simulink model "ES200A_CurrMeas"  (R2013b)
settings: Solver=FixedStepDiscrete  SolverMode=SingleTasking  StartTime=0.0  StopTime=1  FixedStep=0.000125  RelTol=1e-3
values from neighbouring files (symbols this model uses):
  ARCHGLBPRM_2PI_ULS_F32 = DataDict.Constant    [ES200A_CurrMeas_DataDict.m]
  CurrMeasEolGainMax = DataDict.Calibration    [ES200A_CurrMeas_DataDict.m]
  CurrMeasEolGainMin = DataDict.Calibration    [ES200A_CurrMeas_DataDict.m]
  CurrMeasEolGainNrOfSample = DataDict.Calibration    [ES200A_CurrMeas_DataDict.m]
  CurrMeasEolGainNumer = DataDict.Calibration    [ES200A_CurrMeas_DataDict.m]
  CurrMeasEolMaxMotVel = DataDict.Calibration    [ES200A_CurrMeas_DataDict.m]
  CurrMeasEolOffsHiBrdgVltgMin = DataDict.Calibration    [ES200A_CurrMeas_DataDict.m]
  CurrMeasEolOffsHiCmuOffs = DataDict.Calibration    [ES200A_CurrMeas_DataDict.m]
  CurrMeasEolOffsLoCmuOffs = DataDict.Calibration    [ES200A_CurrMeas_DataDict.m]
  CurrMeasEolOffsMax = DataDict.Calibration    [ES200A_CurrMeas_DataDict.m]
  CurrMeasEolOffsMin = DataDict.Calibration    [ES200A_CurrMeas_DataDict.m]
  CurrMeasEolOffsNrOfSample = DataDict.Calibration    [ES200A_CurrMeas_DataDict.m]
  CurrMeasEolTranCntrThd = DataDict.Calibration    [ES200A_CurrMeas_DataDict.m]
  CurrMeasMinRqrdPhaOnTi = DataDict.Calibration    [ES200A_CurrMeas_DataDict.m]
  CurrMeasMotAgCompuDly = DataDict.Calibration    [ES200A_CurrMeas_DataDict.m]
  CurrMeasMotCurrAdcVlyWrmIninMax = DataDict.Calibration    [ES200A_CurrMeas_DataDict.m]
  CurrMeasMotCurrAdcVlyWrmIninMin = DataDict.Calibration    [ES200A_CurrMeas_DataDict.m]
  CurrMeasNtc0x05DFailStep = DataDict.Calibration    [ES200A_CurrMeas_DataDict.m]
  CurrMeasNtc0x05DPassStep = DataDict.Calibration    [ES200A_CurrMeas_DataDict.m]
  CurrMeasNtc0x06DFailStep = DataDict.Calibration    [ES200A_CurrMeas_DataDict.m]
  CurrMeasNtc0x06DPassStep = DataDict.Calibration    [ES200A_CurrMeas_DataDict.m]
  DEGREES30_MOTRAD_F32 = DataDict.Constant    [ES200A_CurrMeas_DataDict.m]
  DIFOFFSRNGCHKMAX_VOLT_F32 = DataDict.Constant    [ES200A_CurrMeas_DataDict.m]
  ELECGLBPRM_IVTRCNT_CNT_U08 = DataDict.ConfigParam    [ES200A_CurrMeas_DataDict.m]
  ELECGLBPRM_STRTUPSTCURRMEASWRMININTESTSTRT_CNT_U08 = DataDict.Constant    [ES200A_CurrMeas_DataDict.m]
  FLTINJ_CURRMEAS_MOTCURRCORRDA = DataDict.Constant    [ES200A_CurrMeas_DataDict.m]
  FLTINJ_CURRMEAS_MOTCURRCORRDD = DataDict.Constant    [ES200A_CurrMeas_DataDict.m]
  FLTINJ_CURRMEAS_TESTOK = DataDict.Constant    [ES200A_CurrMeas_DataDict.m]
  MAXCURRCORRD_AMPR_F32 = DataDict.Constant    [ES200A_CurrMeas_DataDict.m]
  PhaABCMeasdOutOfRng = DataDict.NTC    [ES200A_CurrMeas_DataDict.m]
  PhaDEFMeasOutOfRng = DataDict.NTC    [ES200A_CurrMeas_DataDict.m]
  SysGlbPrmMotPoleCnt = DataDict.ImprtdCal    [ES200A_CurrMeas_DataDict.m]
libraries: simulink x10, FixdToFloat x1
(part 4 of 7)

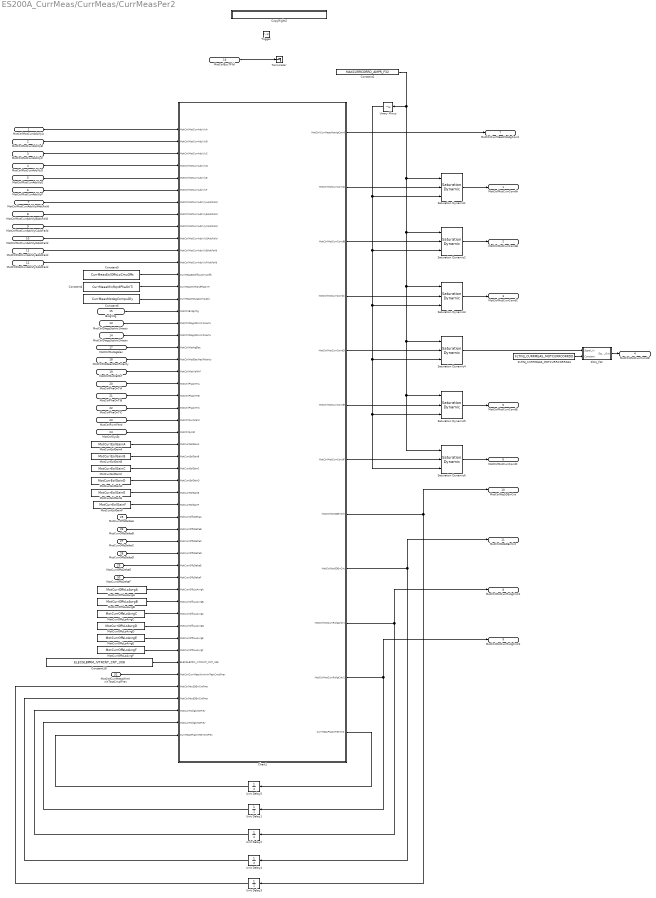
== system ES200A_CurrMeas/CurrMeas/CurrMeasPer2 ==
  MotCtrlMotCurrAdcVlyA : Inport  RequirementInfo={} %GIDa_51523d33_6191_4b88_8694_817dc9ded571
  MotCtrlMotCurrAdcVlyB : Inport  RequirementInfo={} %GIDa_1328ae42_ae96_4bf4_89b7_7635d71eb55f  Port=2
  MotCtrlMotCurrAdcVlyC : Inport  RequirementInfo={} %GIDa_141aa39a_2219_4c7a_8648_7879c9127c56  Port=3
  MotCtrlMotCurrAdcVlyD : Inport  RequirementInfo={} %GIDa_0bb8dbbc_c7c5_4117_b4a1_ced2a35897c9  Port=4
  MotCtrlMotCurrAdcVlyE : Inport  RequirementInfo={} %GIDa_e7be49ef_22f9_4690_b020_08185c31c438  Port=5
  MotCtrlMotCurrAdcVlyF : Inport  RequirementInfo={} %GIDa_885c6b45_efc1_4125_8826_e1fe2f9bfc98  Port=6
  MotCtrlMotCurrAdcVlyAAdcFaild : Inport  RequirementInfo={} %GIDa_d667bfad_9ccb_4ad0_ab64_59c5adeb3cfc  Port=7
  MotCtrlMotCurrAdcVlyBAdcFaild : Inport  RequirementInfo={} %GIDa_614f9520_457f_4a4d_a608_e6a9d7384c30  Port=8
  MotCtrlMotCurrAdcVlyCAdcFaild : Inport  RequirementInfo={} %GIDa_26dea516_d730_426b_b0f7_aef164a4b4a7  Port=9
  MotCtrlMotCurrAdcVlyDAdcFaild : Inport  RequirementInfo={} %GIDa_a9ef4412_4995_4ff8_a712_a0004978e7c0  Port=10
  MotCtrlMotCurrAdcVlyEAdcFaild : Inport  RequirementInfo={} %GIDa_8c5e2e43_d825_49af_8c14_bb63c0e12ba2  Port=11
  MotCtrlMotCurrAdcVlyFAdcFaild : Inport  RequirementInfo={} %GIDa_7ba5334c_0964_494c_9a84_9ee8fa4a837c  Port=12
  MotCtrlDiagcStsIvtr1Inactv : Inport  Port=13
  MotCtrlDiagcStsIvtr2Inactv : Inport  Port=14
  BrdgVltg : Inport  Port=15
  MotCtrlEcuTFild : Inport  RequirementInfo={} %GIDa_37deaa24_f58f_4dab_941a_680d37588f61  Port=16
  MotCtrlMotAgElec : Inport  Port=17
  MotCtrlMotElecMeclPolarity : Inport  Port=18
  MotCtrlMotVelMrf : Inport  Port=19
  MotCtrlPhaOnTiA : Inport  Port=20
  MotCtrlPhaOnTiB : Inport  Port=21
  MotCtrlPhaOnTiC : Inport  Port=22
  MotCtrlPwmPerd : Inport  Port=23
  MotCtrlSysSt : Inport  Port=24
  MotCurrOffsDeltaA : Inport  Port=25
  MotCurrOffsDeltaB : Inport  Port=26
  MotCurrOffsDeltaC : Inport  Port=27
  MotCurrOffsDeltaD : Inport  Port=28
  MotCurrOffsDeltaE : Inport  Port=29
  MotCurrOffsDeltaF : Inport  Port=30
  " MotCtrlCurrMeasWrmIninTestCmplPrev" : Inport  Port=31
  Trigger : TriggerPort  TriggerType=function-call  PortDimensions=1
  Chart1 : Stateflow chart  RequirementInfo={} %GIDa_9666b06e_9e22_4012_a59d_551b4af1f380  TreatAsAtomicUnit=on
  Constant18 : Constant  Value=ELECGLBPRM_IVTRCNT_CNT_U08
  Constant2 : Constant  Value=MAXCURRCORRD_AMPR_F32
  Constant4 : Constant  Value=CurrMeasMinRqrdPhaOnTi
  Constant5 : Constant  Value=CurrMeasEolOffsLoCmuOffs
  Constant6 : Constant  Value=CurrMeasMotAgCompuDly
  CopyRight2 : Subsystem  Description=|  mask(Copyright Information){none=on}
      | Copyright info block.                                               
      |                                                                     
      | Place copyright information at the top of every subsystem in design.
      mask prompts: none "No parameters"
      mask help: Place copyright information at the top of every subsystem in design.
      mask Display:
      | NxtrConf = 'Nexteer Confidential';
      | 
      | sys = bdroot; %handle for the current model ("system")
      | first = get_param(sys,'Created');
      | first = first(end-3:end);  %year is last four digits
      | 
      | last = get_param(sys,'LastModifiedDate');
      | if isempty(last)
      |     last = datestr(now,'yyyy');
      | else
      |     last = last(end-3:end);
      | end
      | 
      | if strcmp(first,last)
      |     fprintf('%s -- Copyright %s Nexteer',NxtrConf,first)
      | else
      |     fprintf('%s -- %s%s- %s Nexteer',NxtrConf,char(169),first,last)
      | end
  FLTINJ_CURRMEAS_MOTCURRCORRDA1 : Constant  Value=FLTINJ_CURRMEAS_MOTCURRCORRDD
  FltInj_f32 : Subsystem  RequirementInfo={'linktype_rmi_doors' '000089bc (/ESG Group/FDD Module Requirements/EA4 Specific/ES200A_CurrMeas)' '#ES200A_267' 'true' 'REQ: ES200A_267' '' } %GIDa_347b8ae7_8767_40c8_a00c_71aafa320d2d  TreatAsAtomicUnit=on  VariantControl=FltInj_sim  mask(Fault_Injection){}
      mask help: Fault Injection is a simulation only block for EA3 programs.
  MotCurrEolGainA : DataStoreRead  DataStoreName=MotCurrEolGainA
  MotCurrEolGainB : DataStoreRead  DataStoreName=MotCurrEolGainB
  MotCurrEolGainC : DataStoreRead  DataStoreName=MotCurrEolGainC
  MotCurrEolGainD : DataStoreRead  DataStoreName=MotCurrEolGainD
  MotCurrEolGainE : DataStoreRead  DataStoreName=MotCurrEolGainE
  MotCurrEolGainF : DataStoreRead  DataStoreName=MotCurrEolGainF
  MotCurrOffsLoAvrgA : DataStoreRead  DataStoreName=MotCurrOffsLoAvrgA
  MotCurrOffsLoAvrgB : DataStoreRead  DataStoreName=MotCurrOffsLoAvrgB
  MotCurrOffsLoAvrgC : DataStoreRead  DataStoreName=MotCurrOffsLoAvrgC
  MotCurrOffsLoAvrgD : DataStoreRead  DataStoreName=MotCurrOffsLoAvrgD
  MotCurrOffsLoAvrgE : DataStoreRead  DataStoreName=MotCurrOffsLoAvrgE
  MotCurrOffsLoAvrgF : DataStoreRead  DataStoreName=MotCurrOffsLoAvrgF
  Saturation Dynamic1 : simulink/Discontinuities/Saturation Dynamic  RequirementInfo={} %GIDa_a678ac9c_94e0_45a6_bd24_feb3ddad182c  OutMin=[]  OutMax=[]  OutDataTypeStr=Inherit: Same as second input  OutDataType=fixdt(1, 16)  OutScaling=2^-10  DoSatur=off
  Saturation Dynamic2 : simulink/Discontinuities/Saturation Dynamic  RequirementInfo={} %GIDa_ad27d5c1_4180_4794_bb6c_e90600e03b36  OutMin=[]  OutMax=[]  OutDataTypeStr=Inherit: Same as second input  OutDataType=fixdt(1, 16)  OutScaling=2^-10  DoSatur=off
  Saturation Dynamic3 : simulink/Discontinuities/Saturation Dynamic  RequirementInfo={} %GIDa_b6946fe3_e777_41d1_91e9_ba0e49afc616  OutMin=[]  OutMax=[]  OutDataTypeStr=Inherit: Same as second input  OutDataType=fixdt(1, 16)  OutScaling=2^-10  DoSatur=off
  Saturation Dynamic4 : simulink/Discontinuities/Saturation Dynamic  RequirementInfo={} %GIDa_eac887ff_7631_462d_b878_5019172b3d55  OutMin=[]  OutMax=[]  OutDataTypeStr=Inherit: Same as second input  OutDataType=fixdt(1, 16)  OutScaling=2^-10  DoSatur=off
  Saturation Dynamic5 : simulink/Discontinuities/Saturation Dynamic  RequirementInfo={} %GIDa_d9181953_bf05_4f89_9278_4fcbc01ab15c  OutMin=[]  OutMax=[]  OutDataTypeStr=Inherit: Same as second input  OutDataType=fixdt(1, 16)  OutScaling=2^-10  DoSatur=off
  Saturation Dynamic6 : simulink/Discontinuities/Saturation Dynamic  RequirementInfo={} %GIDa_4da0401d_6120_4b21_aef3_0a502043331b  OutMin=[]  OutMax=[]  OutDataTypeStr=Inherit: Same as second input  OutDataType=fixdt(1, 16)  OutScaling=2^-10  DoSatur=off
  Terminator : Terminator
  Unary Minus : UnaryMinus
  Unit Delay1 : UnitDelay  SampleTime=-1  StateName=MotCurrRollgCnt2Prev  StateMustResolveToSignalObject=on
      settings: AttributesFormatString=|
      | State Variable:
      | %<StateName>
  Unit Delay2 : UnitDelay  SampleTime=-1  StateName=MotCurrRollgCnt1Prev  StateMustResolveToSignalObject=on
      settings: AttributesFormatString=|
      | State Variable:
      | %<StateName>
  Unit Delay3 : UnitDelay  SampleTime=-1  StateName=MotCtrlNtc5DErrCntPrev  StateMustResolveToSignalObject=on
      settings: AttributesFormatString=|
      | State Variable:
      | %<StateName>
  Unit Delay4 : UnitDelay  SampleTime=-1  StateName=MotCtrlNtc6DErrCntPrev  StateMustResolveToSignalObject=on
      settings: AttributesFormatString=|
      | State Variable:
      | %<StateName>
  Unit Delay5 : UnitDelay  SampleTime=-1  StateName=PhaOnTiErrCntPrev  StateMustResolveToSignalObject=on
      settings: AttributesFormatString=|
      | State Variable:
      | %<StateName>
  MotCtrlMotCurrCorrdA : Outport  RequirementInfo={} %GIDa_be45cc68_c253_4805_9e57_9f0cd86a4b75
  MotCtrlMotCurrCorrdB : Outport  RequirementInfo={} %GIDa_38a03b4c_0b98_4645_8602_2d424e547661  Port=2
  MotCtrlMotCurrCorrdC : Outport  RequirementInfo={} %GIDa_14a10ace_ee81_4ce4_9336_8f01f385929c  Port=3
  MotCtrlMotCurrCorrdD : Outport  RequirementInfo={} %GIDa_2faaf7ab_4344_43ac_a199_98727489f260  Port=4
  MotCtrlMotCurrCorrdE : Outport  RequirementInfo={} %GIDa_8650b4b3_021a_4514_9f56_5151faf8a566  Port=5
  MotCtrlMotCurrCorrdF : Outport  RequirementInfo={} %GIDa_2593a86b_f65b_45be_b765_d74bea967e23  Port=6
  MotCtrlCurrMeasMotAgCorrd : Outport  RequirementInfo={} %GIDa_90a95302_1bff_47e7_a89a_896fae3a575d  Port=7
  MotCtrlMotCurrRollgCntr1 : Outport  RequirementInfo={} %GIDa_aefa170b_455b_48cb_95aa_73c7254f08bd  Port=8
  MotCtrlMotCurrRollgCntr2 : Outport  RequirementInfo={} %GIDa_b45ba8e0_1343_4e05_96b1_238e41ca7131  Port=9
  MotCtrlNtc5DErrCnt : Outport  RequirementInfo={} %GIDa_6d95d8c9_c06f_4998_9e76_5195a73bd44f  Port=10
  MotCtrlNtc6DErrCnt : Outport  RequirementInfo={} %GIDa_f3d2e981_43dc_4e53_81d4_c9088f8342fd  Port=11
  wires:
  MotCtrlEcuTFild/1 -> Terminator/1
  MotCtrlMotCurrAdcVlyAAdcFaild/1 -> Chart1/7(MotCtrlMotCurrAdcVlyAAdcFaild)
  MotCtrlMotCurrAdcVlyBAdcFaild/1 -> Chart1/8(MotCtrlMotCurrAdcVlyBAdcFaild)
  MotCtrlMotCurrAdcVlyDAdcFaild/1 -> Chart1/10(MotCtrlMotCurrAdcVlyDAdcFaild)
  MotCtrlMotCurrAdcVlyFAdcFaild/1 -> Chart1/12(MotCtrlMotCurrAdcVlyFAdcFaild)
  MotCtrlMotCurrAdcVlyEAdcFaild/1 -> Chart1/11(MotCtrlMotCurrAdcVlyEAdcFaild)
  MotCtrlMotCurrAdcVlyCAdcFaild/1 -> Chart1/9(MotCtrlMotCurrAdcVlyCAdcFaild)
  Saturation Dynamic1/1 -> MotCtrlMotCurrCorrdA/1
  FltInj_f32/1(Signal_Out) -> MotCtrlMotCurrCorrdD/1
  FLTINJ_CURRMEAS_MOTCURRCORRDA1/1 -> FltInj_f32/2(Constant)
  Constant4/1 -> Chart1/14(CurrMeasMinRqrdPhaOnTi)
  Constant5/1 -> Chart1/13(CurrMeasEolOffsLoCmuOffs)
  Constant6/1 -> Chart1/15(CurrMeasMotAgCompuDly)
  MotCtrlMotVelMrf/1 -> Chart1/21(MotCtrlMotVelMrf)
  MotCtrlMotElecMeclPolarity/1 -> Chart1/20(MotCtrlMotElecMeclPolarity)
  BrdgVltg/1 -> Chart1/16(MotCtrlBrdgVltg)
  MotCtrlDiagcStsIvtr1Inactv/1 -> Chart1/17(MotCtrlDiagcStsIvtr1Inactv)
  MotCtrlDiagcStsIvtr2Inactv/1 -> Chart1/18(MotCtrlDiagcStsIvtr2Inactv)
  Constant18/1 -> Chart1/45(ELECGLBPRM_IVTRCNT_CNT_U08)
  Unit Delay1/1 -> Chart1/50(MotCurrRollgCnt2Prev)
  Unit Delay2/1 -> Chart1/49(MotCurrRollgCnt1Prev)
  Saturation Dynamic4/1 -> FltInj_f32/1(Signal_In)
  Saturation Dynamic2/1 -> MotCtrlMotCurrCorrdB/1
  Saturation Dynamic3/1 -> MotCtrlMotCurrCorrdC/1
  Saturation Dynamic5/1 -> MotCtrlMotCurrCorrdE/1
  Saturation Dynamic6/1 -> MotCtrlMotCurrCorrdF/1
  Chart1/10(MotCtrlMotCurrRollgCntr1) -> MotCtrlMotCurrRollgCntr1/1, Unit Delay2/1
  Chart1/11(MotCtrlMotCurrRollgCntr2) -> MotCtrlMotCurrRollgCntr2/1, Unit Delay1/1
  Chart1/1(MotCtrlCurrMeasMotAgCorrd) -> MotCtrlCurrMeasMotAgCorrd/1
  MotCurrOffsLoAvrgB/1 -> Chart1/40(MotCurrOffsLoAvrgB)
  MotCurrOffsLoAvrgA/1 -> Chart1/39(MotCurrOffsLoAvrgA)
  MotCurrOffsLoAvrgD/1 -> Chart1/42(MotCurrOffsLoAvrgD)
  MotCurrOffsLoAvrgC/1 -> Chart1/41(MotCurrOffsLoAvrgC)
  MotCurrOffsLoAvrgF/1 -> Chart1/44(MotCurrOffsLoAvrgF)
  MotCurrOffsLoAvrgE/1 -> Chart1/43(MotCurrOffsLoAvrgE)
  MotCurrEolGainF/1 -> Chart1/32(MotCurrEolGainF)
  MotCurrEolGainD/1 -> Chart1/30(MotCurrEolGainD)
  MotCurrEolGainE/1 -> Chart1/31(MotCurrEolGainE)
  MotCurrEolGainB/1 -> Chart1/28(MotCurrEolGainB)
  MotCurrEolGainC/1 -> Chart1/29(MotCurrEolGainC)
  MotCurrEolGainA/1 -> Chart1/27(MotCurrEolGainA)
  MotCurrOffsDeltaD/1 -> Chart1/36(MotCurrOffsDeltaD)
  MotCurrOffsDeltaC/1 -> Chart1/35(MotCurrOffsDeltaC)
  MotCtrlPhaOnTiC/1 -> Chart1/24(MotCtrlPhaOnTiC)
  MotCtrlSysSt/1 -> Chart1/26(MotCtrlSysSt)
  MotCtrlPwmPerd/1 -> Chart1/25(MotCtrlPwmPerd)
  MotCtrlPhaOnTiB/1 -> Chart1/23(MotCtrlPhaOnTiB)
  MotCurrOffsDeltaE/1 -> Chart1/37(MotCurrOffsDeltaE)
  MotCtrlPhaOnTiA/1 -> Chart1/22(MotCtrlPhaOnTiA)
  MotCurrOffsDeltaF/1 -> Chart1/38(MotCurrOffsDeltaF)
  MotCurrOffsDeltaA/1 -> Chart1/33(MotCurrOffsDeltaA)
  MotCurrOffsDeltaB/1 -> Chart1/34(MotCurrOffsDeltaB)
  Unit Delay4/1 -> Chart1/48(MotCtrlNtc6DErrCntPrev)
  Unit Delay3/1 -> Chart1/47(MotCtrlNtc5DErrCntPrev)
  Chart1/9(MotCtrlNtc6DErrCnt) -> MotCtrlNtc6DErrCnt/1, Unit Delay4/1
  Chart1/8(MotCtrlNtc5DErrCnt) -> MotCtrlNtc5DErrCnt/1, Unit Delay3/1
  " MotCtrlCurrMeasWrmIninTestCmplPrev"/1 -> Chart1/46(MotCtrlCurrMeasWrmIninTestCmplPrev)
  Unit Delay5/1 -> Chart1/51(CurrMeasPhaOnTiErrCntPrev)
  Chart1/12(CurrMeasPhaOnTiErrCnt) -> Unit Delay5/1
  Constant2/1 -> Saturation Dynamic3/1, Saturation Dynamic6/1, Saturation Dynamic5/1, Saturation Dynamic4/1, Saturation Dynamic2/1, Saturation Dynamic1/1, Unary Minus/1
  Unary Minus/1 -> Saturation Dynamic3/3, Saturation Dynamic6/3, Saturation Dynamic5/3, Saturation Dynamic4/3, Saturation Dynamic2/3, Saturation Dynamic1/3
  Chart1/2(MotCtrlMotCurrCorrdA) -> Saturation Dynamic1/2
  Chart1/3(MotCtrlMotCurrCorrdB) -> Saturation Dynamic2/2
  Chart1/4(MotCtrlMotCurrCorrdC) -> Saturation Dynamic3/2
  Chart1/5(MotCtrlMotCurrCorrdD) -> Saturation Dynamic4/2
  Chart1/6(MotCtrlMotCurrCorrdE) -> Saturation Dynamic5/2
  Chart1/7(MotCtrlMotCurrCorrdF) -> Saturation Dynamic6/2
  MotCtrlMotAgElec/1 -> Chart1/19(MotCtrlMotAgElec)
  MotCtrlMotCurrAdcVlyE/1 -> Chart1/5(MotCtrlMotCurrAdcVlyE)
  MotCtrlMotCurrAdcVlyD/1 -> Chart1/4(MotCtrlMotCurrAdcVlyD)
  MotCtrlMotCurrAdcVlyB/1 -> Chart1/2(MotCtrlMotCurrAdcVlyB)
  MotCtrlMotCurrAdcVlyC/1 -> Chart1/3(MotCtrlMotCurrAdcVlyC)
  MotCtrlMotCurrAdcVlyF/1 -> Chart1/6(MotCtrlMotCurrAdcVlyF)
  MotCtrlMotCurrAdcVlyA/1 -> Chart1/1(MotCtrlMotCurrAdcVlyA)

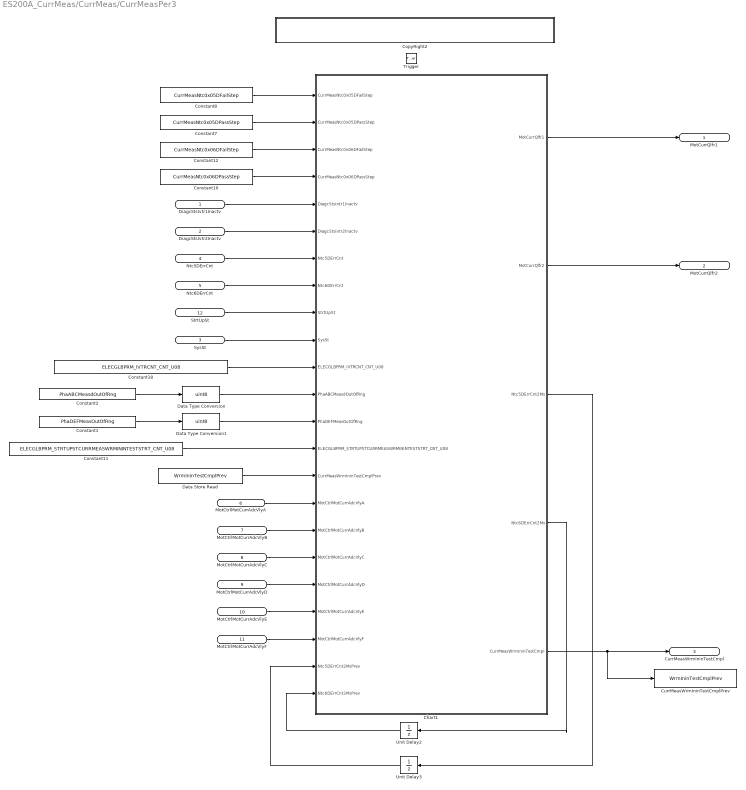
== system ES200A_CurrMeas/CurrMeas/CurrMeasPer3 ==
  DiagcStsIvtr1Inactv : Inport  RequirementInfo={} %GIDa_3f2b24ca_5e64_4642_910e_ca50d78da245
  DiagcStsIvtr2Inactv : Inport  RequirementInfo={} %GIDa_b1a5f59d_5a54_42de_8529_fc0d027b3ef3  Port=2
  SysSt : Inport  RequirementInfo={} %GIDa_ebc52ed6_1f51_43d3_a6da_39b6b9940c04  Port=3  OutDataTypeStr=single
  Ntc5DErrCnt : Inport  RequirementInfo={} %GIDa_ffc53944_d65d_4434_9c9b_5bfc70525927  Port=4  OutDataTypeStr=uint16
  Ntc6DErrCnt : Inport  RequirementInfo={} %GIDa_365cbd76_0dca_48e8_96f7_4dd33cc79fcb  Port=5  OutDataTypeStr=uint16
  MotCtrlMotCurrAdcVlyA : Inport  RequirementInfo={} %GIDa_7bf3cbd7_2538_4e8a_a22d_abe526b19335  Port=6
  MotCtrlMotCurrAdcVlyB : Inport  RequirementInfo={} %GIDa_7698553c_2590_423a_a37b_077079574e3f  Port=7
  MotCtrlMotCurrAdcVlyC : Inport  RequirementInfo={} %GIDa_493e93c2_e8a9_4c58_98a0_ce115796497b  Port=8
  MotCtrlMotCurrAdcVlyD : Inport  RequirementInfo={} %GIDa_dcf6e783_ea97_45aa_b2df_a8b40ffd71d9  Port=9
  MotCtrlMotCurrAdcVlyE : Inport  RequirementInfo={} %GIDa_a4c14b22_ad3d_4d49_8f67_e25589a32bce  Port=10
  MotCtrlMotCurrAdcVlyF : Inport  RequirementInfo={} %GIDa_1f7c68b9_6400_46f6_8cd6_6a391c1de49a  Port=11
  StrtUpSt : Inport  RequirementInfo={} %GIDa_1f30c06a_d58b_4090_b4a6_84109da18cdc  Port=12  OutDataTypeStr=single
  Trigger : TriggerPort  TriggerType=function-call  PortDimensions=1
  Chart1 : Stateflow chart  TreatAsAtomicUnit=on
  Constant1 : Constant  Value=PhaDEFMeasOutOfRng
  Constant10 : Constant  Value=CurrMeasNtc0x06DPassStep
  Constant11 : Constant  Value=ELECGLBPRM_STRTUPSTCURRMEASWRMININTESTSTRT_CNT_U08
  Constant12 : Constant  Value=CurrMeasNtc0x06DFailStep
  Constant18 : Constant  Value=ELECGLBPRM_IVTRCNT_CNT_U08
  Constant2 : Constant  Value=PhaABCMeasdOutOfRng
  Constant7 : Constant  Value=CurrMeasNtc0x05DPassStep
  Constant8 : Constant  Value=CurrMeasNtc0x05DFailStep
  CopyRight2 : Subsystem  Description=|  mask(Copyright Information){none=on}
      | Copyright info block.                                               
      |                                                                     
      | Place copyright information at the top of every subsystem in design.
      mask prompts: none "No parameters"
      mask help: Place copyright information at the top of every subsystem in design.
      mask Display:
      | NxtrConf = 'Nexteer Confidential';
      | 
      | sys = bdroot; %handle for the current model ("system")
      | first = get_param(sys,'Created');
      | first = first(end-3:end);  %year is last four digits
      | 
      | last = get_param(sys,'LastModifiedDate');
      | if isempty(last)
      |     last = datestr(now,'yyyy');
      | else
      |     last = last(end-3:end);
      | end
      | 
      | if strcmp(first,last)
      |     fprintf('%s -- Copyright %s Nexteer',NxtrConf,first)
      | else
      |     fprintf('%s -- %s%s- %s Nexteer',NxtrConf,char(169),first,last)
      | end
  CurrMeasWrmIninTestCmplPrev : DataStoreWrite  RequirementInfo={} %GIDa_56301e73_d1a5_44f0_9c00_c95c5be8192d  DataStoreName=WrmIninTestCmplPrev  DataStoreElements=WrmIninTestCmplPrev
  Data Store Read : DataStoreRead  DataStoreName=WrmIninTestCmplPrev  DataStoreElements=WrmIninTestCmplPrev
  Data Type Conversion : DataTypeConversion  OutDataTypeStr=uint8
  Data Type Conversion1 : DataTypeConversion  OutDataTypeStr=uint8
  Unit Delay2 : UnitDelay  SampleTime=-1  StateName=Ntc6DErrCnt2MilliSecPrev  StateMustResolveToSignalObject=on
      settings: AttributesFormatString=|
      | State Variable:
      | %<StateName>
  Unit Delay3 : UnitDelay  SampleTime=-1  StateName=Ntc5DErrCnt2MilliSecPrev  StateMustResolveToSignalObject=on
      settings: AttributesFormatString=|
      | State Variable:
      | %<StateName>
  MotCurrQlfr1 : Outport  RequirementInfo={} %GIDa_97d5bfb1_2351_42dd_b658_023a6d8f5aa1
  MotCurrQlfr2 : Outport  RequirementInfo={} %GIDa_e2da2e04_5849_4da3_a687_01333d2236a2  Port=2
  CurrMeasWrmIninTestCmpl : Outport  RequirementInfo={} %GIDa_b01ce9a2_2e51_43fa_ab76_6aeab0dbecf7  Port=3
  wires:
  Constant10/1 -> Chart1/4(CurrMeasNtc0x06DPassStep)
  Constant7/1 -> Chart1/2(CurrMeasNtc0x05DPassStep)
  Constant12/1 -> Chart1/3(CurrMeasNtc0x06DFailStep)
  Constant8/1 -> Chart1/1(CurrMeasNtc0x05DFailStep)
  DiagcStsIvtr1Inactv/1 -> Chart1/5(DiagcStsIvtr1Inactv)
  DiagcStsIvtr2Inactv/1 -> Chart1/6(DiagcStsIvtr2Inactv)
  Ntc5DErrCnt/1 -> Chart1/7(Ntc5DErrCnt)
  Ntc6DErrCnt/1 -> Chart1/8(Ntc6DErrCnt)
  Constant18/1 -> Chart1/11(ELECGLBPRM_IVTRCNT_CNT_U08)
  Constant11/1 -> Chart1/14(ELECGLBPRM_STRTUPSTCURRMEASWRMININTESTSTRT_CNT_U08)
  SysSt/1 -> Chart1/10(SysSt)
  Chart1/3(Ntc5DErrCnt2Ms) -> Unit Delay3/1
  Chart1/4(Ntc6DErrCnt2Ms) -> Unit Delay2/1
  Chart1/5(CurrMeasWrmIninTestCmpl) -> CurrMeasWrmIninTestCmpl/1, CurrMeasWrmIninTestCmplPrev/1
  Chart1/1(MotCurrQlfr1) -> MotCurrQlfr1/1
  Chart1/2(MotCurrQlfr2) -> MotCurrQlfr2/1
  Unit Delay2/1 -> Chart1/23(Ntc6DErrCnt2MsPrev)
  Unit Delay3/1 -> Chart1/22(Ntc5DErrCnt2MsPrev)
  Data Store Read/1 -> Chart1/15(CurrMeasWrmIninTestCmplPrev)
  Constant1/1 -> Data Type Conversion1/1
  Constant2/1 -> Data Type Conversion/1
  Data Type Conversion/1 -> Chart1/12(PhaABCMeasdOutOfRng)
  Data Type Conversion1/1 -> Chart1/13(PhaDEFMeasOutOfRng)
  MotCtrlMotCurrAdcVlyA/1 -> Chart1/16(MotCtrlMotCurrAdcVlyA)
  MotCtrlMotCurrAdcVlyB/1 -> Chart1/17(MotCtrlMotCurrAdcVlyB)
  MotCtrlMotCurrAdcVlyC/1 -> Chart1/18(MotCtrlMotCurrAdcVlyC)
  MotCtrlMotCurrAdcVlyD/1 -> Chart1/19(MotCtrlMotCurrAdcVlyD)
  MotCtrlMotCurrAdcVlyE/1 -> Chart1/20(MotCtrlMotCurrAdcVlyE)
  MotCtrlMotCurrAdcVlyF/1 -> Chart1/21(MotCtrlMotCurrAdcVlyF)
  StrtUpSt/1 -> Chart1/9(StrtUpSt)

== system ES200A_CurrMeas/CurrMeas/FltInj_f32 ==
  note: This block requires no modification by FDD author.
      |
      | This block does not actually simulate any fault injection.  It is simply a pass-thru.
      |
      | The Constant port (#2) simply terminates its signal, but we are trying to force the FDD author
      | to properly use the FltInjectionLocType enumeration in FDD model.
  note: EA4.x Fault Injection
  Signal_In : Inport
  Constant : Inport  Port=2
  CopyRight2 : Subsystem  Description=|  mask(Copyright Information){none=on}
      | Copyright info block.                                               
      |                                                                     
      | Place copyright information at the top of every subsystem in design.
      mask prompts: none "No parameters"
      mask help: Place copyright information at the top of every subsystem in design.
      mask Display:
      | NxtrConf = 'Nexteer Confidential';
      | 
      | sys = bdroot; %handle for the current model ("system")
      | first = get_param(sys,'Created');
      | first = first(end-3:end);  %year is last four digits
      | 
      | last = get_param(sys,'LastModifiedDate');
      | if isempty(last)
      |     last = datestr(now,'yyyy');
      | else
      |     last = last(end-3:end);
      | end
      | 
      | if strcmp(first,last)
      |     fprintf('%s -- Copyright %s Nexteer',NxtrConf,first)
      | else
      |     fprintf('%s -- %s%s- %s Nexteer',NxtrConf,char(169),first,last)
      | end
  Terminator : Terminator
  Signal_Out : Outport
  wires:
  Signal_In/1 -> Signal_Out/1
  Constant/1 -> Terminator/1

== system ES200A_CurrMeas/CurrMeas/CurrMeasEolGainReq/CopyRight2 ==

== system ES200A_CurrMeas/CurrMeas/CurrMeasEolGainStsReq/CopyRight2 ==

== system ES200A_CurrMeas/CurrMeas/CurrMeasEolOffsReq/CopyRight2 ==

== system ES200A_CurrMeas/CurrMeas/CurrMeasEolOffsStsReq/CopyRight2 ==

== system ES200A_CurrMeas/CurrMeas/CurrMeasGainReadReq/CopyRight2 ==

== system ES200A_CurrMeas/CurrMeas/CurrMeasGainWrReq/CopyRight2 ==

== system ES200A_CurrMeas/CurrMeas/CurrMeasGainWrReq/IF ==
  CurrMeasMotCurrGainA_ArgIn : Inport  RequirementInfo={} %GIDa_87b59b63_6625_4c38_a995_a430fafe0129  OutDataTypeStr=single
  CurrMeasMotCurrGainB_ArgIn : Inport  RequirementInfo={} %GIDa_77d3c118_6d5d_4a6d_bf43_acbab5c55649  Port=2  OutDataTypeStr=single
  CurrMeasMotCurrGainC_ArgIn : Inport  RequirementInfo={} %GIDa_50760476_4eb4_4fe6_81a8_acdf6cdf4679  Port=3  OutDataTypeStr=single
  CurrMeasMotCurrGainD_ArgIn : Inport  RequirementInfo={} %GIDa_e8971956_e66c_49cd_b063_7f3e149dc0e1  Port=4  OutDataTypeStr=single
  CurrMeasMotCurrGainE_ArgIn : Inport  RequirementInfo={} %GIDa_9ee4b377_1ed8_4e03_968c_c6f167646a4a  Port=5  OutDataTypeStr=single
  CurrMeasMotCurrGainF_ArgIn : Inport  RequirementInfo={} %GIDa_824e1cae_8662_42c6_b5bf_076ba0b66ddf  Port=6  OutDataTypeStr=single
  Action Port : ActionPort  ActionType=then
  Constant14 : Constant  OutDataTypeStr=single
  CurrMeasEolGainCalSet : DataStoreWrite  RequirementInfo={'linktype_rmi_doors' '000089bc (/ESG Group/FDD Module Requirements/EA4 Specific/ES200A_CurrMeas)' '#ES200A_291' 'true' 'REQ: ES200A_291' '' } %GIDa_e0bf40b3_7bb6_4054_b3a0_3f5c2964ab0c  DataStoreName=CurrMeasEolGainCalSet  DataStoreElements=CurrMeasEolGainCalSet.CurrMeasMotCurrEolGainA#CurrMeasEolGainCalSet.CurrMeasMotCurrEolGainB#CurrMeasEolGainCalSet.CurrMeasMotCurrEolGainC#CurrMeasEolGainCalSet.CurrMeasMotCurrEolGainD#CurrMeasEolGainCalSet.CurrMeasMotCurrEolGainE#CurrMeasEolGainCalSet.CurrMeasMotCurrEolGainF
  CurrMeasEolGainCalSet_SetRamBlockStatus : Subsystem  RequirementInfo={'linktype_rmi_doors' '000089bc (/ESG Group/FDD Module Requirements/EA4 Specific/ES200A_CurrMeas)' '#ES200A_291' 'true' 'REQ: ES200A_291' '' } %GIDa_5922b5b3_8031_4b5e_94b1_30094195ff33  TreatAsAtomicUnit=on
  Positive Response : Constant  Value=0
  CurrMeasGainWrReqSts : Outport  RequirementInfo={} %GIDa_db75dea6_25d1_4b9e_bf3d_93caa7994694
  wires:
  Constant14/1 -> CurrMeasEolGainCalSet_SetRamBlockStatus/1("BlockChanged ")
  CurrMeasMotCurrGainA_ArgIn/1 -> CurrMeasEolGainCalSet/1
  CurrMeasMotCurrGainB_ArgIn/1 -> CurrMeasEolGainCalSet/2
  CurrMeasMotCurrGainD_ArgIn/1 -> CurrMeasEolGainCalSet/4
  CurrMeasMotCurrGainE_ArgIn/1 -> CurrMeasEolGainCalSet/5
  CurrMeasMotCurrGainC_ArgIn/1 -> CurrMeasEolGainCalSet/3
  CurrMeasMotCurrGainF_ArgIn/1 -> CurrMeasEolGainCalSet/6
  Positive Response/1 -> CurrMeasGainWrReqSts/1

== system ES200A_CurrMeas/CurrMeas/CurrMeasGainWrReq/else  ==
  Action Port : ActionPort  ActionType=else
  Negative Response : Constant
  CurrMeasGainWrReqSts : Outport  RequirementInfo={} %GIDa_7081d4be_b2eb_437d_b738_c85b18ebe99c
  wires:
  Negative Response/1 -> CurrMeasGainWrReqSts/1

== system ES200A_CurrMeas/CurrMeas/CurrMeasInit1/CopyRight2 ==

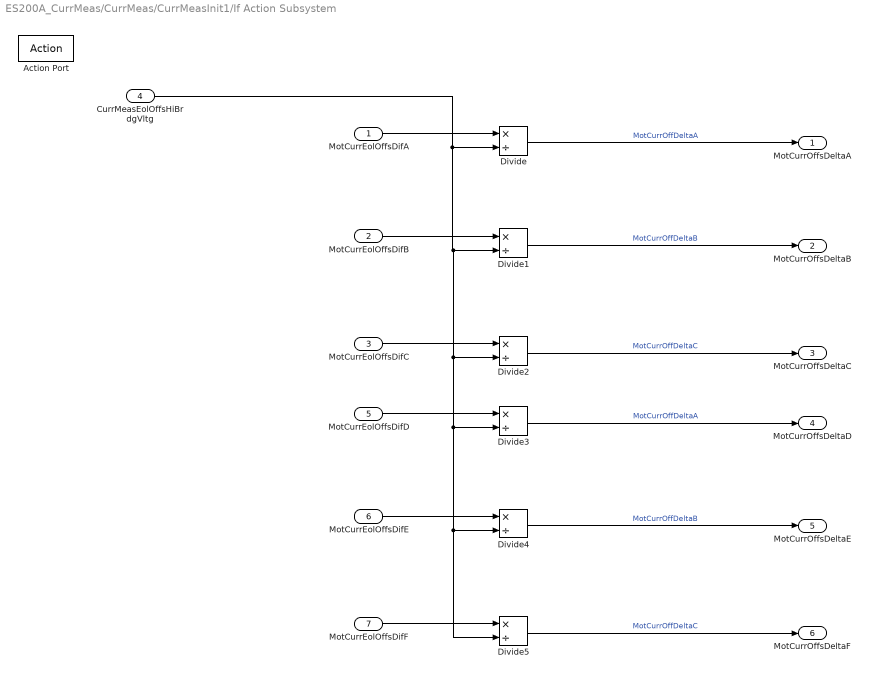
== system ES200A_CurrMeas/CurrMeas/CurrMeasInit1/If Action Subsystem ==
  MotCurrEolOffsDifA : Inport  OutDataTypeStr=single
  MotCurrEolOffsDifB : Inport  Port=2  OutDataTypeStr=single
  MotCurrEolOffsDifC : Inport  Port=3  OutDataTypeStr=single
  CurrMeasEolOffsHiBrdgVltg : Inport  Port=4  OutDataTypeStr=single
  MotCurrEolOffsDifD : Inport  Port=5  OutDataTypeStr=single
  MotCurrEolOffsDifE : Inport  Port=6  OutDataTypeStr=single
  MotCurrEolOffsDifF : Inport  Port=7  OutDataTypeStr=single
  Action Port : ActionPort  ActionType=then
  Divide{,1..5} (6 alike) : Product  Inputs=*/
  MotCurrOffsDeltaA : Outport  OutDataTypeStr=single
  MotCurrOffsDeltaB : Outport  Port=2  OutDataTypeStr=single
  MotCurrOffsDeltaC : Outport  Port=3  OutDataTypeStr=single
  MotCurrOffsDeltaD : Outport  Port=4  OutDataTypeStr=single
  MotCurrOffsDeltaE : Outport  Port=5  OutDataTypeStr=single
  MotCurrOffsDeltaF : Outport  Port=6  OutDataTypeStr=single
  wires:
  MotCurrEolOffsDifA/1 -> Divide/1
  MotCurrEolOffsDifB/1 -> Divide1/1
  MotCurrEolOffsDifC/1 -> Divide2/1
  Divide/1 -> MotCurrOffsDeltaA/1  "MotCurrOffDeltaA"
  Divide1/1 -> MotCurrOffsDeltaB/1  "MotCurrOffDeltaB"
  Divide2/1 -> MotCurrOffsDeltaC/1  "MotCurrOffDeltaC"
  MotCurrEolOffsDifD/1 -> Divide3/1
  MotCurrEolOffsDifE/1 -> Divide4/1
  MotCurrEolOffsDifF/1 -> Divide5/1
  CurrMeasEolOffsHiBrdgVltg/1 -> Divide5/2, Divide4/2, Divide3/2, Divide2/2, Divide1/2, Divide/2
  Divide3/1 -> MotCurrOffsDeltaD/1  "MotCurrOffDeltaA"
  Divide4/1 -> MotCurrOffsDeltaE/1  "MotCurrOffDeltaB"
  Divide5/1 -> MotCurrOffsDeltaF/1  "MotCurrOffDeltaC"

== system ES200A_CurrMeas/CurrMeas/CurrMeasInit1/If Action Subsystem1 ==
  Action Port : ActionPort  ActionType=else
  Constant{,1..5} (6 alike) : Constant  Value=0  OutDataTypeStr=single
  MotCurrOffsDeltaA : Outport
  MotCurrOffsDeltaB : Outport  Port=2
  MotCurrOffsDeltaC : Outport  Port=3
  MotCurrOffsDeltaD : Outport  Port=4
  MotCurrOffsDeltaE : Outport  Port=5
  MotCurrOffsDeltaF : Outport  Port=6
  wires:
  Constant2/1 -> MotCurrOffsDeltaC/1  "MotCurrOffDeltaC"
  Constant1/1 -> MotCurrOffsDeltaB/1  "MotCurrOffDeltaB"
  Constant/1 -> MotCurrOffsDeltaA/1  "MotCurrOffDeltaA"
  Constant3/1 -> MotCurrOffsDeltaD/1
  Constant4/1 -> MotCurrOffsDeltaE/1
  Constant5/1 -> MotCurrOffsDeltaF/1

== system ES200A_CurrMeas/CurrMeas/CurrMeasOffsReadReq/CopyRight2 ==

== system ES200A_CurrMeas/CurrMeas/CurrMeasOffsWrReq/CopyRight2 ==

== stateflow chart ES200A_CurrMeas/CurrMeas/CurrMeasPer1/Gain Calibration/GainStateMachine/SetNtcSts/SetNtcSts/ISO Fault Debounce Design ==
  note: Pass Loop
  note: Fail Loop
  note: 
  note: NTCSTS_PASSD           (0)
      | NTCSTS_FAILD             (1)
      | NTCSTS_PREPASSD   (2)
      | NTCSTS_PREFAILD     (3)
      |
      | SIGQLFR_NORES        (0)
      | SIGQLFR_PASSD         (1)
      | SIGQLFR_FAILD           (2)
  note: Condition not present for 2nd Transition for first connective junction in PassLoop. Changed it to [NtcSts ==2]
  note: Swapped conditional transition([SvcClr ==1]
      | {ErrAcc = 0;
      | Qualifier =0;
      | }) from 2nd priority to 1st
  (default) -> (junction 89)
  (junction 89) -> (junction 95) [order 1] : [NtcSts ==3]
  (junction 89) -> (junction 93) [order 2] : [NtcSts ==2]
  (junction 89) -> (junction 141) [order 3] : [NtcSts ==1]
      | { ErrAcc = 32767;
      | Qualifier =2;
      |  }
  (junction 89) -> (junction 141) [order 4] : [NtcSts ==0]
      | { ErrAcc = -32768;
      | Qualifier=1;
      | }
  (junction 95) -> (junction 103) [order 2]
  (junction 95) -> (junction 111) [order 1] : [ErrAcc <=0]
      | {ErrAcc = DebStep;}
  (junction 93) -> (junction 123) [order 2] : {
      | ErrAcc = ErrAcc - DebStep;
      | }
  (junction 93) -> (junction 123) [order 1] : [(ErrAcc - DebStep) <= -32768]
      | { ErrAcc = -32768;
      | Qualifier=1;
      | }
  (junction 103) -> (junction 111) [order 1] : [(ErrAcc + DebStep) <32767]
      | {ErrAcc = ErrAcc + DebStep;}
  (junction 103) -> (junction 111) [order 2] : {ErrAcc = 32767;
      | Qualifier =2;}
  (junction 123) -> (junction 141)
  (junction 111) -> (junction 141)
  (junction 141) -> (junction 159) [order 2]
  (junction 141) -> (junction 159) [order 1] : [SvcClr ==1]
      | {ErrAcc = 0;
      | Qualifier =0;
      | }
  data: NtcSts input uint8; Qualifier output uint8; DebStep input int32; ErrAcc local single; SvcClr input

== stateflow chart ES200A_CurrMeas/CurrMeas/CurrMeasPer1/Offset Calibration/Offset State Machine/SetNtcSts/SetNtcSts/ISO Fault Debounce Design ==
  note: Pass Loop
  note: Fail Loop
  note: 
  note: NTCSTS_PASSD           (0)
      | NTCSTS_FAILD             (1)
      | NTCSTS_PREPASSD   (2)
      | NTCSTS_PREFAILD     (3)
      |
      | SIGQLFR_NORES        (0)
      | SIGQLFR_PASSD         (1)
      | SIGQLFR_FAILD           (2)
  note: Condition not present for 2nd Transition for first connective junction in PassLoop. Changed it to [NtcSts ==2]
  note: Swapped conditional transition([SvcClr ==1]
      | {ErrAcc = 0;
      | Qualifier =0;
      | }) from 2nd priority to 1st
  (default) -> (junction 89)
  (junction 89) -> (junction 95) [order 1] : [NtcSts ==3]
  (junction 89) -> (junction 93) [order 2] : [NtcSts ==2]
  (junction 89) -> (junction 141) [order 3] : [NtcSts ==1]
      | { ErrAcc = 32767;
      | Qualifier =2;
      |  }
  (junction 89) -> (junction 141) [order 4] : [NtcSts ==0]
      | { ErrAcc = -32768;
      | Qualifier=1;
      | }
  (junction 95) -> (junction 103) [order 2]
  (junction 95) -> (junction 111) [order 1] : [ErrAcc <=0]
      | {ErrAcc = DebStep;}
  (junction 93) -> (junction 123) [order 2] : {
      | ErrAcc = ErrAcc - DebStep;
      | }
  (junction 93) -> (junction 123) [order 1] : [(ErrAcc - DebStep) <= -32768]
      | { ErrAcc = -32768;
      | Qualifier=1;
      | }
  (junction 103) -> (junction 111) [order 1] : [(ErrAcc + DebStep) <32767]
      | {ErrAcc = ErrAcc + DebStep;}
  (junction 103) -> (junction 111) [order 2] : {ErrAcc = 32767;
      | Qualifier =2;}
  (junction 123) -> (junction 141)
  (junction 111) -> (junction 141)
  (junction 141) -> (junction 159) [order 2]
  (junction 141) -> (junction 159) [order 1] : [SvcClr ==1]
      | {ErrAcc = 0;
      | Qualifier =0;
      | }
  data: NtcSts input uint8; Qualifier output uint8; DebStep input int32; ErrAcc local single; SvcClr input

== system ES200A_CurrMeas/CurrMeas/CurrMeasOffsWrReq/IF ==
  CurrMeasEolOffsHiBrdgVltg_ArgIn : Inport  RequirementInfo={} %GIDa_812a1a2f_8d9b_493f_8d38_cf559d2e2313  OutDataTypeStr=single
  CurrMeasMotCurrOffsDifA_ArgIn : Inport  RequirementInfo={} %GIDa_620df217_6d23_4379_b697_2438223fdb1e  Port=2  OutDataTypeStr=single
  CurrMeasMotCurrOffsLoAvrgA_ArgIn : Inport  RequirementInfo={} %GIDa_fbdbb2e3_d8ba_4172_b27f_3be627a5f176  Port=3  OutDataTypeStr=single
  CurrMeasMotCurrOffsLoAvrgB_ArgIn : Inport  RequirementInfo={} %GIDa_4342fbfc_d634_403b_9b29_d8803beea53e  Port=4  OutDataTypeStr=single
  CurrMeasMotCurrOffsLoAvrgC_ArgIn : Inport  RequirementInfo={} %GIDa_1155a904_daa1_442b_9b3a_76183cfeb8de  Port=5  OutDataTypeStr=single
  CurrMeasMotCurrOffsLoAvrgD_ArgIn : Inport  RequirementInfo={} %GIDa_b5928048_b518_475c_bd85_7d449910b834  Port=6  OutDataTypeStr=single
  CurrMeasMotCurrOffsLoAvrgE_ArgIn : Inport  RequirementInfo={} %GIDa_2f4f2a2a_6567_449e_882d_b458829ff196  Port=7  OutDataTypeStr=single
  CurrMeasMotCurrOffsLoAvrgF_ArgIn : Inport  RequirementInfo={} %GIDa_a7fe6648_99b2_41ba_8ec9_da3c20c2e7af  Port=8  OutDataTypeStr=single
  CurrMeasMotCurrOffsDifB_ArgIn : Inport  RequirementInfo={} %GIDa_17cf677d_9485_4eb6_bf0d_5d95365246ca  Port=9  OutDataTypeStr=single
  CurrMeasMotCurrOffsDifC_ArgIn : Inport  RequirementInfo={} %GIDa_8d171d0b_2ff9_462a_9ae6_84a29f9d80d8  Port=10  OutDataTypeStr=single
  CurrMeasMotCurrOffsDifD_ArgIn : Inport  RequirementInfo={} %GIDa_84414505_75c9_4dd9_ba80_d7374193ac56  Port=11  OutDataTypeStr=single
  CurrMeasMotCurrOffsDifE_ArgIn : Inport  RequirementInfo={} %GIDa_d54e2248_e490_46ca_9d40_ef0ba9a5a858  Port=12  OutDataTypeStr=single
  CurrMeasMotCurrOffsDifF_ArgIn : Inport  RequirementInfo={} %GIDa_15e5f242_fd24_4678_b9cf_ed0d82bfd499  Port=13  OutDataTypeStr=single
  Action Port : ActionPort  ActionType=then
  Constant14 : Constant  OutDataTypeStr=single
  CurrMeasEolOffsCalSet : DataStoreWrite  RequirementInfo={'linktype_rmi_doors' '000089bc (/ESG Group/FDD Module Requirements/EA4 Specific/ES200A_CurrMeas)' '#ES200A_280' 'true' 'REQ: ES200A_280' '' } %GIDa_65bd6eae_4bc4_46b4_a91f_58c4237add93  DataStoreName=CurrMeasEolOffsCalSet  DataStoreElements=CurrMeasEolOffsCalSet.CurrMeasEolOffsHiBrdgVltg#CurrMeasEolOffsCalSet.CurrMeasMotCurrEolOffsDifA#CurrMeasEolOffsCalSet.CurrMeasMotCurrEolOffsDifB#CurrMeasEolOffsCalSet.CurrMeasMotCurrEolOffsDifC#CurrMeasEolOffsCalSet.CurrMeasMotCurrEolOffsDifD#CurrMeasEolOffsCalSet.CurrMeasMotCurrEolOffsDifE#CurrMeasEolOffsCalSet.CurrMeasMotCurrEolOffsDifF#CurrMeasEolOffsCalSet.CurrMeasMotCurrOffsLoAvrgA#CurrMeasEolOffsCalSet.CurrMeasMotCurrOffsLoAvrgB#CurrMeasEolOffsCalSet.CurrMeasMotCurrOffsLoAvrgC#CurrMeasEolOffsCalSet.CurrMeasMotCurrOffsLoAvrgD#CurrMeasEolOffsCalSet.CurrMeasMotCurrOffsLoAvrgE#CurrMeasEolOffsCalSet.CurrMeasMotCurrOffsLoAvrgF
  CurrMeasEolOffsCalSet_SetRamBlockStatus : Subsystem  RequirementInfo={'linktype_rmi_doors' '000089bc (/ESG Group/FDD Module Requirements/EA4 Specific/ES200A_CurrMeas)' '#ES200A_280' 'true' 'REQ: ES200A_280' '' } %GIDa_fdbbe63c_7b7e_430e_a45c_f1a2eec3b0d3  TreatAsAtomicUnit=on
  Positive Response : Constant  Value=0
  CurrMeasOffsWrReqSts : Outport  RequirementInfo={} %GIDa_d6bd7840_4b1f_429e_aa0e_09addb50176a
  wires:
  CurrMeasMotCurrOffsDifB_ArgIn/1 -> CurrMeasEolOffsCalSet/3
  CurrMeasMotCurrOffsDifA_ArgIn/1 -> CurrMeasEolOffsCalSet/2
  CurrMeasMotCurrOffsLoAvrgC_ArgIn/1 -> CurrMeasEolOffsCalSet/10
  CurrMeasMotCurrOffsLoAvrgD_ArgIn/1 -> CurrMeasEolOffsCalSet/11
  CurrMeasMotCurrOffsLoAvrgF_ArgIn/1 -> CurrMeasEolOffsCalSet/13
  CurrMeasMotCurrOffsDifF_ArgIn/1 -> CurrMeasEolOffsCalSet/7
  CurrMeasMotCurrOffsDifC_ArgIn/1 -> CurrMeasEolOffsCalSet/4
  CurrMeasMotCurrOffsDifE_ArgIn/1 -> CurrMeasEolOffsCalSet/6
  CurrMeasMotCurrOffsLoAvrgB_ArgIn/1 -> CurrMeasEolOffsCalSet/9
  CurrMeasMotCurrOffsDifD_ArgIn/1 -> CurrMeasEolOffsCalSet/5
  CurrMeasMotCurrOffsLoAvrgA_ArgIn/1 -> CurrMeasEolOffsCalSet/8
  CurrMeasMotCurrOffsLoAvrgE_ArgIn/1 -> CurrMeasEolOffsCalSet/12
  Constant14/1 -> CurrMeasEolOffsCalSet_SetRamBlockStatus/1("BlockChanged ")
  CurrMeasEolOffsHiBrdgVltg_ArgIn/1 -> CurrMeasEolOffsCalSet/1
  Positive Response/1 -> CurrMeasOffsWrReqSts/1

== system ES200A_CurrMeas/CurrMeas/CurrMeasOffsWrReq/else  ==
  Action Port : ActionPort  ActionType=else
  Negative Response : Constant
  CurrMeasOffsWrReqSts : Outport  RequirementInfo={} %GIDa_bbade129_568d_4f6a_aeaa_1c5484c89fdb
  wires:
  Negative Response/1 -> CurrMeasOffsWrReqSts/1

== system ES200A_CurrMeas/CurrMeas/CurrMeasPer1/CopyRight2 ==

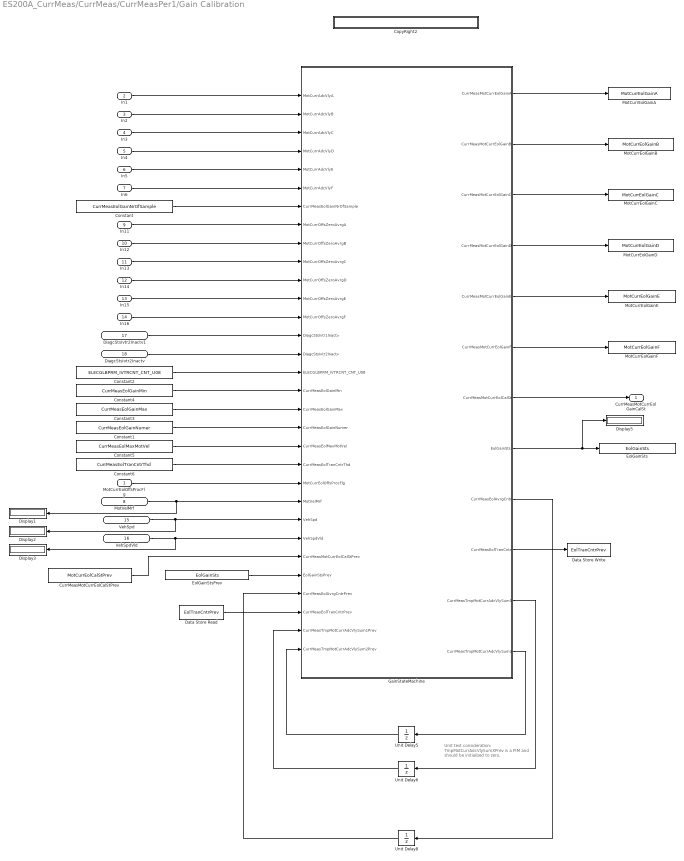
== system ES200A_CurrMeas/CurrMeas/CurrMeasPer1/Gain Calibration ==
  note: Unit test consideration:
      | TmpMotCurrAdcVlySumXPrev is a PIM
      | and should be initialized to zero.
  MotCurrEolOffsProcFlg : Inport
  In1 : Inport  Port=2
  In2 : Inport  Port=3
  In3 : Inport  Port=4
  In4 : Inport  Port=5
  In5 : Inport  Port=6
  In6 : Inport  Port=7
  MotVelMrf : Inport  RequirementInfo={} %GIDa_a7b78662_7cf0_48ed_9f87_08134d024c78  Port=8  OutDataTypeStr=single
  In11 : Inport  Port=9
  In12 : Inport  Port=10
  In13 : Inport  Port=11
  In14 : Inport  Port=12
  In15 : Inport  Port=13
  In16 : Inport  Port=14
  VehSpd : Inport  RequirementInfo={} %GIDa_c841d099_fc23_4afc_9dd2_bf4d1285ca82  Port=15
  VehSpdVld : Inport  RequirementInfo={} %GIDa_a5c49bc6_dd19_4849_b83d_4c3bf1157af9  Port=16  OutDataTypeStr=single
  DiagcStsIvtr2Inactv1 : Inport  RequirementInfo={} %GIDa_8700043e_90fa_4116_85b4_a3555476b354  Port=17
  DiagcStsIvtr2Inactv : Inport  RequirementInfo={} %GIDa_425966d8_d289_4e11_9dbb_57044454bfa8  Port=18
  Constant : Constant  Value=CurrMeasEolGainNrOfSample
  Constant1 : Constant  Value=CurrMeasEolGainNumer
  Constant2 : Constant  Value=ELECGLBPRM_IVTRCNT_CNT_U08  OutDataTypeStr=uint8
  Constant3 : Constant  Value=CurrMeasEolGainMax
  Constant4 : Constant  Value=CurrMeasEolGainMin
  Constant5 : Constant  Value=CurrMeasEolMaxMotVel
  Constant6 : Constant  Value=CurrMeasEolTranCntrThd
  CopyRight2 : Subsystem  Description=|  mask(Copyright Information){none=on}
      | Copyright info block.                                               
      |                                                                     
      | Place copyright information at the top of every subsystem in design.
      mask prompts: none "No parameters"
      mask help: Place copyright information at the top of every subsystem in design.
      mask Display:
      | NxtrConf = 'Nexteer Confidential';
      | 
      | sys = bdroot; %handle for the current model ("system")
      | first = get_param(sys,'Created');
      | first = first(end-3:end);  %year is last four digits
      | 
      | last = get_param(sys,'LastModifiedDate');
      | if isempty(last)
      |     last = datestr(now,'yyyy');
      | else
      |     last = last(end-3:end);
      | end
      | 
      | if strcmp(first,last)
      |     fprintf('%s -- Copyright %s Nexteer',NxtrConf,first)
      | else
      |     fprintf('%s -- %s%s- %s Nexteer',NxtrConf,char(169),first,last)
      | end
  CurrMeasMotCurrEolCalStPrev : DataStoreRead  DataStoreName=MotCurrEolCalStPrev  DataStoreElements=MotCurrEolCalStPrev
  Data Store Read : DataStoreRead  DataStoreName=EolTranCntrPrev
  Data Store Write : DataStoreWrite  DataStoreName=EolTranCntrPrev
  Display{1..3,5} (4 alike) : Display
  EolGainSts : DataStoreWrite  DataStoreName=EolGainSts
  EolGainStsPrev : DataStoreRead  DataStoreName=EolGainSts  DataStoreElements=EolGainSts
  GainStateMachine : Stateflow chart  RequirementInfo={'linktype_rmi_doors' '000089bc (/ESG Group/FDD Module Requirements/EA4 Specific/ES200A_CurrMeas)' '#ES200A_174' 'true' 'REQ: ES200A_174' '' } %GIDa_289e43b1_cfe4_41ba_9e49_3210dfe736ba  TreatAsAtomicUnit=on
  MotCurrEolGainA : DataStoreWrite  RequirementInfo={} %GIDa_13893fc7_c204_439f_bffc_cfe8ef3246c0  DataStoreName=MotCurrEolGainA
  MotCurrEolGainB : DataStoreWrite  RequirementInfo={} %GIDa_bd072951_11b3_473d_b14d_56675fe847ea  DataStoreName=MotCurrEolGainB
  MotCurrEolGainC : DataStoreWrite  RequirementInfo={} %GIDa_85f7aa39_8d03_4989_9937_397e0bbdc0c3  DataStoreName=MotCurrEolGainC
  MotCurrEolGainD : DataStoreWrite  RequirementInfo={} %GIDa_b5965ed2_4a8c_4234_8376_930d7494d8ae  DataStoreName=MotCurrEolGainD
  MotCurrEolGainE : DataStoreWrite  RequirementInfo={} %GIDa_5641d146_2eac_4d29_ad9c_8f8105bea573  DataStoreName=MotCurrEolGainE
  MotCurrEolGainF : DataStoreWrite  RequirementInfo={} %GIDa_25d2bb4a_a4ab_4b72_9cc3_33d4fd2a8c29  DataStoreName=MotCurrEolGainF
  Unit Delay5 : UnitDelay  SampleTime=-1  StateName=TmpMotCurrAdcVlySum2Prev  StateMustResolveToSignalObject=on
      settings: AttributesFormatString=|
      | State Variable:
      | %<StateName>
  Unit Delay6 : UnitDelay  SampleTime=-1  StateName=TmpMotCurrAdcVlySum1Prev  StateMustResolveToSignalObject=on
      settings: AttributesFormatString=|
      | State Variable:
      | %<StateName>
  Unit Delay8 : UnitDelay  SampleTime=-1  StateName=GainEolAvrgCntrPrev  StateMustResolveToSignalObject=on
      settings: AttributesFormatString=|
      | State Variable:
      | %<StateName>
  CurrMeasMotCurrEolGainCalSt : Outport  OutDataTypeStr=Enum: MotCurrEolCalSt2
  wires:
  GainStateMachine/1(CurrMeasMotCurrEolGainA) -> MotCurrEolGainA/1
  GainStateMachine/2(CurrMeasMotCurrEolGainB) -> MotCurrEolGainB/1
  GainStateMachine/3(CurrMeasMotCurrEolGainC) -> MotCurrEolGainC/1
  GainStateMachine/5(CurrMeasMotCurrEolGainE) -> MotCurrEolGainE/1
  GainStateMachine/6(CurrMeasMotCurrEolGainF) -> MotCurrEolGainF/1
  GainStateMachine/4(CurrMeasMotCurrEolGainD) -> MotCurrEolGainD/1
  GainStateMachine/8(EolGainSts) -> Display5/1, EolGainSts/1
  GainStateMachine/7(CurrMeasMotCurrEolCalSt) -> CurrMeasMotCurrEolGainCalSt/1
  In14/1 -> GainStateMachine/11(MotCurrOffsZeroAvrgD)
  In15/1 -> GainStateMachine/12(MotCurrOffsZeroAvrgE)
  In16/1 -> GainStateMachine/13(MotCurrOffsZeroAvrgF)
  In11/1 -> GainStateMachine/8(MotCurrOffsZeroAvrgA)
  In12/1 -> GainStateMachine/9(MotCurrOffsZeroAvrgB)
  In13/1 -> GainStateMachine/10(MotCurrOffsZeroAvrgC)
  Constant5/1 -> GainStateMachine/20(CurrMeasEolMaxMotVel)
  Constant6/1 -> GainStateMachine/21(CurrMeasEolTranCntrThd)
  Constant3/1 -> GainStateMachine/18(CurrMeasEolGainMax)
  Constant1/1 -> GainStateMachine/19(CurrMeasEolGainNumer)
  Constant4/1 -> GainStateMachine/17(CurrMeasEolGainMin)
  MotVelMrf/1 -> Display1/1, GainStateMachine/23(MotVelMrf)
  EolGainStsPrev/1 -> GainStateMachine/27(EolGainStsPrev)
  VehSpdVld/1 -> Display3/1, GainStateMachine/25(VehSpdVld)
  VehSpd/1 -> Display2/1, GainStateMachine/24(VehSpd)
  CurrMeasMotCurrEolCalStPrev/1 -> GainStateMachine/26(CurrMeasMotCurrEolCalStPrev)
  MotCurrEolOffsProcFlg/1 -> GainStateMachine/22(MotCurrEolOffsProcFlg)
  GainStateMachine/9(CurrMeasEolAvrgCntr) -> Unit Delay8/1
  Unit Delay8/1 -> GainStateMachine/28(CurrMeasEolAvrgCntrPrev)
  GainStateMachine/11(CurrMeasTmpMotCurrAdcVlySum1) -> Unit Delay6/1
  Unit Delay6/1 -> GainStateMachine/30(CurrMeasTmpMotCurrAdcVlySum1Prev)
  GainStateMachine/12(CurrMeasTmpMotCurrAdcVlySum2) -> Unit Delay5/1
  Unit Delay5/1 -> GainStateMachine/31(CurrMeasTmpMotCurrAdcVlySum2Prev)
  Constant/1 -> GainStateMachine/7(CurrMeasEolGainNrOfSample)
  In4/1 -> GainStateMachine/4(MotCurrAdcVlyD)
  In3/1 -> GainStateMachine/3(MotCurrAdcVlyC)
  In1/1 -> GainStateMachine/1(MotCurrAdcVlyA)
  In6/1 -> GainStateMachine/6(MotCurrAdcVlyF)
  In5/1 -> GainStateMachine/5(MotCurrAdcVlyE)
  In2/1 -> GainStateMachine/2(MotCurrAdcVlyB)
  Constant2/1 -> GainStateMachine/16(ELECGLBPRM_IVTRCNT_CNT_U08)
  DiagcStsIvtr2Inactv1/1 -> GainStateMachine/14(DiagcStsIvtr1Inactv)
  DiagcStsIvtr2Inactv/1 -> GainStateMachine/15(DiagcStsIvtr2Inactv)
  GainStateMachine/10(CurrMeasEolTranCntr) -> Data Store Write/1
  Data Store Read/1 -> GainStateMachine/29(CurrMeasEolTranCntrPrev)
